simulink model "MotorController3"  (Simulink 10.1)
settings: Solver=ode5  StartTime=0.0  StopTime=100  FixedStep=5e-6  RelTol=1e-4  EnableMultiTasking=on
undefined symbols (not defined in the file): sigbuilder_block
libraries: simulink x5
settings Model: Creator=mf  LastModifiedBy=Lukas Bilal  SimulationMode=accelerator  ExtModeAutoUpdateStatusClock=off
settings Model: ModifiedHistory=|
  | Original Modell stammt von Martin Fränzle, Universität Oldenburg.
  | Erweiterung durch Stefan Disch, Universität Freiburg
settings DataIOCC: LimitDataPoints=on  SignalLoggingSaveFormat=ModelDataLogs  SaveOutput=off  SignalLogging=off  DSMLogging=off  SaveTime=off  SignalLoggingName=sigsOut
settings OptimizationCC: BooleanDataType=off  ExpressionDepthLimit=2147483647  InitFltsAndDblsToZero=on  SimCompilerOptimization=on
settings DebuggingCC: SaveWithParameterizedLinksMsg=none  SignalResolutionControl=TryResolveAllWithWarning  MultiTaskDSMMsg=warning  MultiTaskCondExecSysMsg=none  FcnCallInpInsideContextMsg=warning  StateNameClashWarn=warning
settings HardwareCC: TargetUnknown=on
settings SFSimCC: SimParseCustomCode=off
settings GRTTargetCC: TargetFcnLib=ansi_tfl_tmw.mat  ModelReferenceCompliant=off  MatFileLogging=off

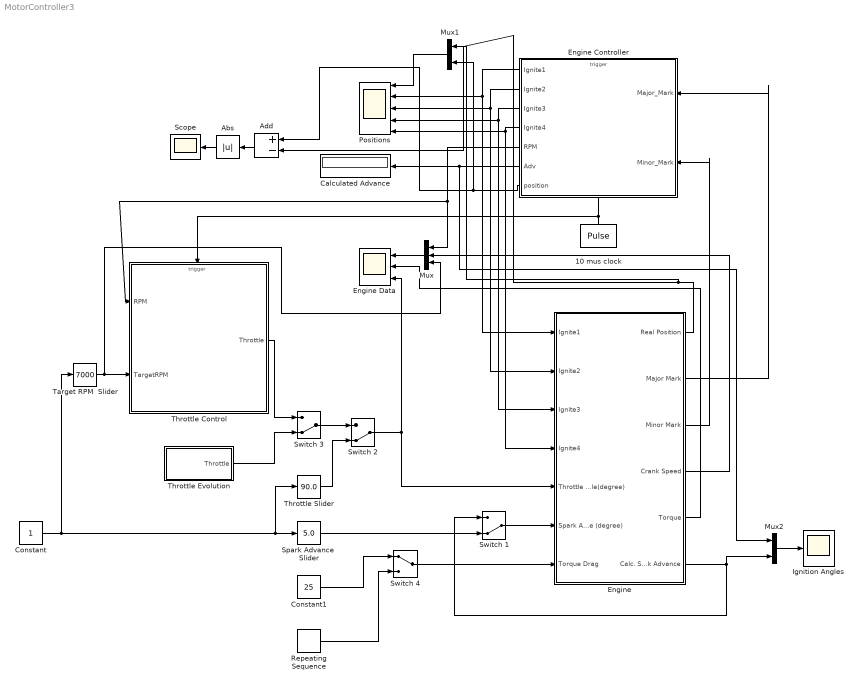
== system MotorController3 ==
  10 mus clock : DiscretePulseGenerator  PulseType=Time based  Period=1e-5  PulseWidth=50
  Abs : Abs
  Add : Sum  Inputs=+-
  Calculated Advance : Display
  Constant : Constant
  Constant1 : Constant  Value=25
  Engine : Subsystem
  Engine Controller : Stateflow chart  TreatAsAtomicUnit=on
  Engine Data : Scope  NumInputPorts=3
  Ignition Angles : Scope
  Mux : Mux  Inputs=3
  Mux1 : Mux  Inputs=2
  Mux2 : Mux  Inputs=2
  Positions : Scope  NumInputPorts=5
  Repeating Sequence : simulink/Sources/Repeating Sequence  rep_seq_t=[0 1 2 3 4 5 6]  rep_seq_y=[20 40 60 80 40 0 20]
  Scope : Scope
  Spark Advance  Slider : simulink/Math Operations/Slider Gain  gain=5.0  low=-15  high=60
  Switch 1 : ManualSwitch  CurrentSetting=0
  Switch 2 : ManualSwitch  CurrentSetting=0
  Switch 3 : ManualSwitch  CurrentSetting=0
  Switch 4 : ManualSwitch
  Target RPM  Slider : simulink/Math Operations/Slider Gain  gain=7000  low=800  high=7000
  Throttle Control : Stateflow chart  TreatAsAtomicUnit=on
  Throttle Evolution : Subsystem  Tag=STV Subsys  LoadFcn=sigbuilder_block('load');  StartFcn=sigbuilder_block('start');  StopFcn=sigbuilder_block('stop');  ClipboardFcn=sigbuilder_block('clipboard');  mask(Sigbuilder block){tuvar=[0:10]}
      mask help: Simulink:masks:SigbuilderBlock_MD
      mask init:
      | if ~strcmp(get_param(bdroot(gcbh),'SimulationStatus'),'stopped') tuvar = sigbuilder_block('maskInit'); end
      settings: CopyFcn=sigbuilder_block('copy');  DeleteFcn=sigbuilder_block('delete');  ModelCloseFcn=sigbuilder_block('modelClose');  PreSaveFcn=sigbuilder_block('preSave');  PauseFcn=sigbuilder_block('pause')  ContinueFcn=sigbuilder_block('continue')  NameChangeFcn=sigbuilder_block('namechange');  OpenFcn=sigbuilder_block('open',[54.75 146.25 550.5 390.75 ]);  CloseFcn=sigbuilder_block('close');
      mask Display: plot(0, 0, 100, 100,[2, 2, 32, 32, 2], [68, 8, 8, 68, 68],[32, 2], [38, 38], [32, 19, 2],[53, 60, 44], [32, 17, 17, 2],[16, 16, 31, 31]);txt = getActiveGroup(gcbh);text(2, 100, txt,'verticalAlignment', 'top');
  Throttle Slider : simulink/Math Operations/Slider Gain  gain=90.0  low=0  high=90
  wires:
  Engine Controller/3(Ignite3) -> Engine/3(Ignite3), Positions/4
  Engine Controller/2(Ignite2) -> Engine/2(Ignite2), Positions/3
  Engine Controller/1(Ignite1) -> Engine/1(Ignite1), Positions/2
  Engine Controller/4(Ignite4) -> Engine/4(Ignite4), Positions/5
  10 mus clock/1 -> Engine Controller/Trigger, Throttle Control/Trigger
  Engine Controller/5(RPM) -> Throttle Control/1(RPM), Mux/1
  Engine Controller/7(position) -> Mux1/2, Add/1
  Mux1/1 -> Positions/1
  Engine Controller/6(Adv) -> Calculated Advance/1, Mux2/1
  Switch 2/1 -> Engine Data/3, Engine/5(Throttle Angle(degree))
  Constant/1 -> Spark Advance  Slider/1, Throttle Slider/1, Target RPM  Slider/1
  Throttle Slider/1 -> Switch 2/2
  Spark Advance  Slider/1 -> Switch 1/2
  Mux2/1 -> Ignition Angles/1
  Mux/1 -> Engine Data/1
  Switch 3/1 -> Switch 2/1
  Throttle Evolution/1(Throttle) -> Switch 3/2
  Throttle Control/1(Throttle) -> Switch 3/1
  Target RPM  Slider/1 -> Throttle Control/2(TargetRPM), Mux/3
  Constant1/1 -> Switch 4/1
  Repeating Sequence/1 -> Switch 4/2
  Engine/6(" Calc. Spark Advance") -> Switch 1/1, Mux2/2
  Switch 1/1 -> Engine/6(Spark Advance (degree))
  Switch 4/1 -> Engine/7(Torque Drag)
  Engine/1(Real Position) -> Mux1/1, Add/2
  Engine/2(Major Mark) -> Engine Controller/1(Major_Mark)
  Engine/3(Minor Mark) -> Engine Controller/2(Minor_Mark)
  Engine/4(Crank Speed) -> Mux/2
  Engine/5(Torque) -> Engine Data/2
  Abs/1 -> Scope/1
  Add/1 -> Abs/1

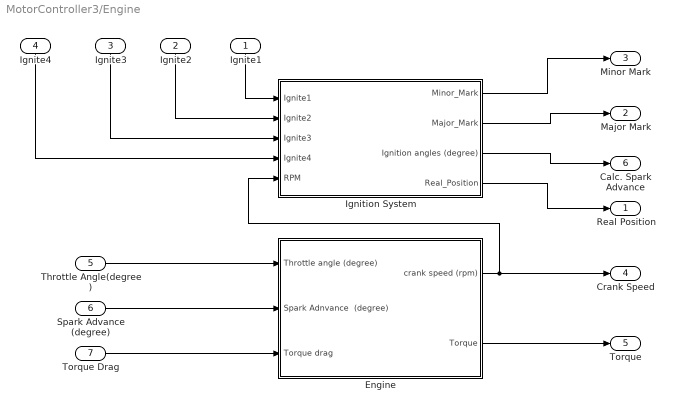
== system MotorController3/Engine ==
  Ignite1 : Inport
  Ignite2 : Inport  Port=2
  Ignite3 : Inport  Port=3
  Ignite4 : Inport  Port=4
  Throttle Angle(degree) : Inport  Port=5
  Spark Advance (degree) : Inport  Port=6
  Torque Drag : Inport  Port=7
  Engine : Subsystem
  Ignition System : Subsystem
  Real Position : Outport
  Major Mark : Outport  Port=2
  Minor Mark : Outport  Port=3
  Crank Speed : Outport  Port=4
  Torque : Outport  Port=5
  " Calc. Spark Advance" : Outport  Port=6
  wires:
  Ignite3/1 -> Ignition System/3(Ignite3)
  Ignite4/1 -> Ignition System/4(Ignite4)
  Ignite1/1 -> Ignition System/1(Ignite1)
  Ignite2/1 -> Ignition System/2(Ignite2)
  Throttle Angle(degree)/1 -> Engine/1(Throttle angle (degree))
  Engine/1(crank speed (rpm)) -> Ignition System/5(RPM), Crank Speed/1
  Ignition System/1(Minor_Mark) -> Minor Mark/1
  Ignition System/2(Major_Mark) -> Major Mark/1
  Ignition System/3(Ignition angles (degree)) -> " Calc. Spark Advance"/1
  Ignition System/4(Real_Position) -> Real Position/1
  Spark Advance (degree)/1 -> Engine/2(Spark Adnvance  (degree))
  Engine/2(Torque) -> Torque/1
  Torque Drag/1 -> Engine/3(Torque drag)

== system MotorController3/Throttle Evolution ==
  Demux : Demux  Tag=STV Demux  Outputs=1
      settings: DisplayOption=none
  FromWs : FromWorkspace  Tag=STV FromWs  VariableName=tuvar  SigBuilderData=DataTag0  VnvData=DataTag1
      SigBuilderData=|
      | common.afterFinalStr = 'Extrapolate'
      | common.sampleTime = 0
      | dataSet.timeRange = [0 14]
      | dataSet.name = 'Group 1'
      | sbobj.Groups.Name = 'Group 1'
      | sbobj.Groups.Signals.Name = 'Throttle'
      | sbobj.Groups.Signals.XData = [0 0.4 1.4 2.4 2.8 3.4 3.8 4.4 5.8 7 8 9.8 12 13.2 14]
      | sbobj.Groups.Signals.YData = [0.2 10 90.2 90 0.2 0.2 90.2 11.8 11.4 26.4 39.8 40.2 40.8 0 0]
      | sbobj.Groups.TimeRange = [0 14]
  Throttle : Outport  Tag=STV Outport
  wires:
  Demux/1 -> Throttle/1
  FromWs/1 -> Demux/1

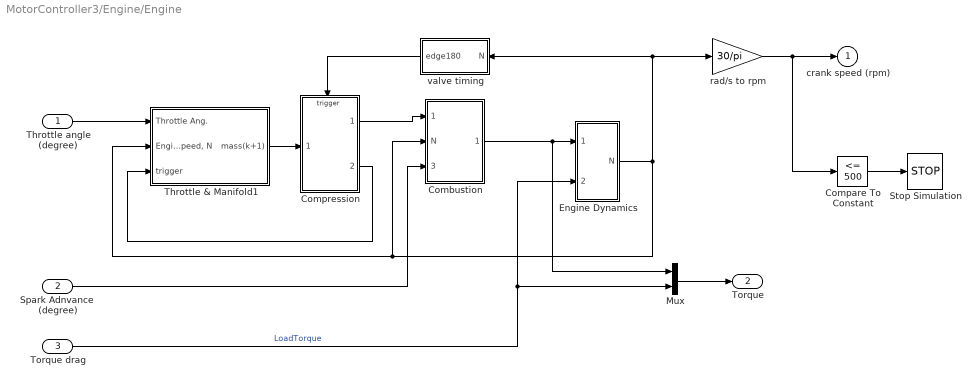
== system MotorController3/Engine/Engine ==
  Throttle angle (degree) : Inport  OutMin=0  OutMax=90  OutDataTypeStr=double
  Spark Adnvance  (degree) : Inport  Port=2
  Torque drag : Inport  Port=3  OutDataTypeStr=double
  Combustion : Subsystem
  Compare To Constant : simulink/Logic and Bit Operations/Compare To Constant  relop=<=  const=500  OutDataTypeStr=boolean
  Compression : Subsystem  TreatAsAtomicUnit=on
  Engine Dynamics : Subsystem
  Mux : Mux  Inputs=2
  Stop Simulation : Stop
  Throttle & Manifold1 : Subsystem
  rad/s to rpm : Gain  Gain=30/pi  SaturateOnIntegerOverflow=on  OutDataTypeStr=Inherit: Same as input  ParamDataTypeStr=Inherit: Same as input
  valve timing : Subsystem
  crank speed (rpm) : Outport  InitialOutput=0
  Torque : Outport  Port=2
  wires:
  valve timing/1(edge180) -> Compression/Trigger
  Compression/2(trigger) -> Throttle & Manifold1/3(trigger)
  Engine Dynamics/1(N) -> valve timing/1(N), rad/s to rpm/1, Throttle & Manifold1/2("Engine Speed, N"), Combustion/2(N)
  Compression/1(mass(k)) -> Combustion/1(Air Charge)
  Combustion/1(Torque) -> Engine Dynamics/1(Teng), Mux/1
  Mux/1 -> Torque/1
  Torque drag/1 -> Engine Dynamics/2(Tload), Mux/2  "LoadTorque"
  Throttle & Manifold1/1(mass(k+1)) -> Compression/1(mass(k+1))
  Throttle angle (degree)/1 -> Throttle & Manifold1/1(Throttle Ang.)
  rad/s to rpm/1 -> crank speed (rpm)/1, Compare To Constant/1
  Spark Adnvance  (degree)/1 -> Combustion/3(Spark Advance)
  Compare To Constant/1 -> Stop Simulation/1

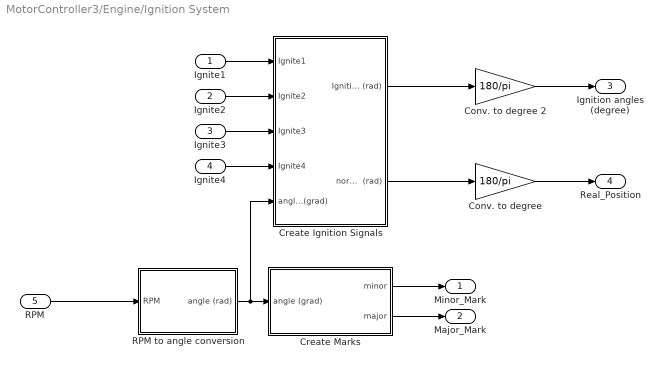
== system MotorController3/Engine/Ignition System ==
  Ignite1 : Inport  OutDataTypeStr=boolean
  Ignite2 : Inport  Port=2  OutDataTypeStr=boolean
  Ignite3 : Inport  Port=3  OutDataTypeStr=boolean
  Ignite4 : Inport  Port=4  OutDataTypeStr=boolean
  RPM : Inport  Port=5
  Conv. to degree : Gain  Gain=180/pi  SaturateOnIntegerOverflow=on  OutDataTypeStr=Inherit: Same as input  ParamDataTypeStr=Inherit: Same as input
  Conv. to degree 2 : Gain  Gain=180/pi  SaturateOnIntegerOverflow=on  OutDataTypeStr=Inherit: Same as input  ParamDataTypeStr=Inherit: Same as input
  Create Ignition Signals : Subsystem
  Create Marks : Subsystem
  RPM to angle conversion : Subsystem
  Minor_Mark : Outport
  Major_Mark : Outport  Port=2
  Ignition angles (degree) : Outport  Port=3
  Real_Position : Outport  Port=4
  wires:
  Create Marks/2(major) -> Major_Mark/1
  Create Marks/1(minor) -> Minor_Mark/1
  Ignite1/1 -> Create Ignition Signals/1(Ignite1)
  Ignite2/1 -> Create Ignition Signals/2(Ignite2)
  Ignite3/1 -> Create Ignition Signals/3(Ignite3)
  Ignite4/1 -> Create Ignition Signals/4(Ignite4)
  Create Ignition Signals/2(normalized angle  (rad)) -> Conv. to degree/1
  Create Ignition Signals/1(Ignition Advance  Angle (rad)) -> Conv. to degree 2/1
  RPM to angle conversion/1(angle (rad)) -> Create Marks/1(angle (grad)), Create Ignition Signals/5(angle (grad))
  Conv. to degree/1 -> Real_Position/1
  Conv. to degree 2/1 -> Ignition angles (degree)/1
  RPM/1 -> RPM to angle conversion/1(RPM)

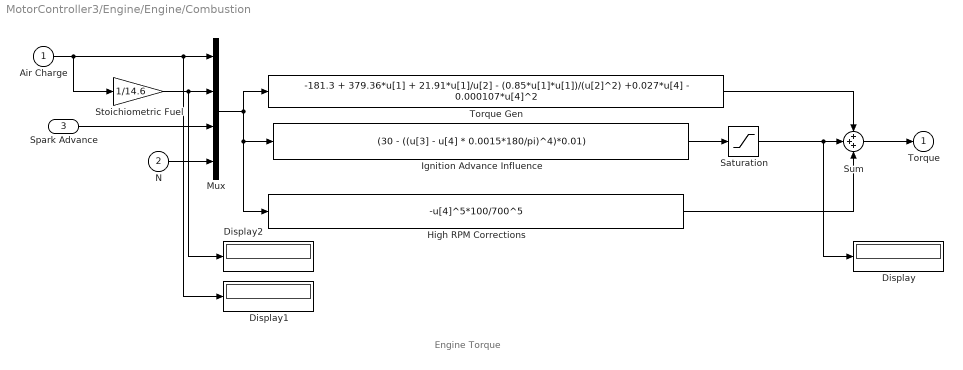
== system MotorController3/Engine/Engine/Combustion ==
  note: Engine Torque
  Air Charge : Inport
  N : Inport  Port=2
  Spark Advance : Inport  Port=3
  Display : Display
  Display1 : Display
  Display2 : Display
  High RPM Corrections : Fcn  Expr=-u[4]^5*100/700^5
  Ignition Advance Influence : Fcn  Expr=(30 - ((u[3] - u[4] * 0.0015*180/pi)^4)*0.01)
  Mux : Mux
  Saturation : Saturate  UpperLimit=150  LowerLimit=-150
  Stoichiometric Fuel : Gain  Gain=1/14.6  SaturateOnIntegerOverflow=on  OutDataTypeStr=Inherit: Same as input  ParamDataTypeStr=Inherit: Same as input
  Sum : Sum  Inputs=+++  InputSameDT=on  SaturateOnIntegerOverflow=on  OutDataTypeStr=Inherit: Same as first input
  Torque Gen : Fcn  Expr=-181.3 + 379.36*u[1] + 21.91*u[1]/u[2] - (0.85*u[1]*u[1])/(u[2]^2) +0.027*u[4] - 0.000107*u[4]^2
  Torque : Outport  InitialOutput=0
  wires:
  Sum/1 -> Torque/1
  Torque Gen/1 -> Sum/1
  Mux/1 -> Torque Gen/1, Ignition Advance Influence/1, High RPM Corrections/1
  Air Charge/1 -> Stoichiometric Fuel/1, Mux/1, Display1/1
  N/1 -> Mux/4
  Spark Advance/1 -> Mux/3
  Stoichiometric Fuel/1 -> Mux/2, Display2/1
  Ignition Advance Influence/1 -> Saturation/1
  High RPM Corrections/1 -> Sum/3
  Saturation/1 -> Sum/2, Display/1

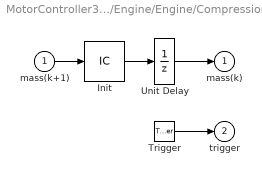
== system MotorController3/Engine/Engine/Compression ==
  mass(k+1) : Inport
  Trigger : TriggerPort  TriggerType=either  VariantControl=(inherit)  ShowOutputPort=on
  Init : InitialCondition  Value=0.152
  Unit Delay : UnitDelay  InitialCondition=0.152  SampleTime=-1  HasFrameUpgradeWarning=on
  mass(k) : Outport  InitialOutput=0.152
  trigger : Outport  Port=2  InitialOutput=-1
  wires:
  Trigger/1 -> trigger/1
  Unit Delay/1 -> mass(k)/1
  mass(k+1)/1 -> Init/1
  Init/1 -> Unit Delay/1

== system MotorController3/Engine/Engine/Engine Dynamics ==
  Teng : Inport
  Tload : Inport  Port=2
  "Inverse Inertia, 1/J" : Gain  Gain=1/0.15  SaturateOnIntegerOverflow=on  OutDataTypeStr=Inherit: Same as input  ParamDataTypeStr=Inherit: Same as input
  Sum : Sum  Inputs=+-  InputSameDT=on  SaturateOnIntegerOverflow=on  OutDataTypeStr=Inherit: Same as first input
  w = T/J w0 = 83.78 rad/s = 800 RPM : Integrator  InitialCondition=83.78
  N : Outport  InitialOutput=0
  wires:
  Tload/1 -> Sum/2
  Teng/1 -> Sum/1
  Sum/1 -> "Inverse Inertia, 1/J"/1
  w = T/J w0 = 83.78 rad/s = 800 RPM/1 -> N/1
  "Inverse Inertia, 1/J"/1 -> w = T/J w0 = 83.78 rad/s = 800 RPM/1

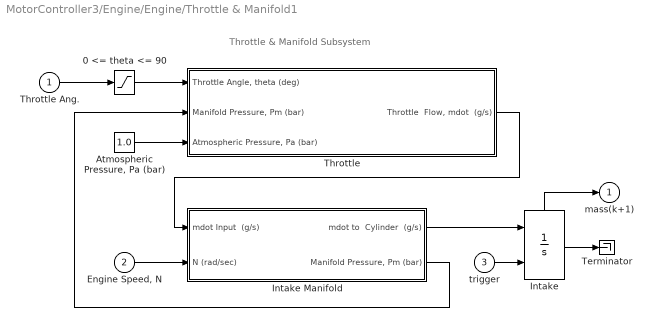
== system MotorController3/Engine/Engine/Throttle & Manifold1 ==
  note: Throttle & Manifold Subsystem
  Throttle Ang. : Inport
  "Engine Speed, N" : Inport  Port=2
  trigger : Inport  Port=3
  0 <= theta <= 90 : Saturate  UpperLimit=90  LowerLimit=0
  "Atmospheric Pressure, Pa (bar)" : Constant  Value=1.0
  Intake : Integrator  ExternalReset=either  ShowStatePort=on
  Intake Manifold : Subsystem
  Terminator : Terminator
  Throttle : Subsystem
  mass(k+1) : Outport  InitialOutput=0
  wires:
  0 <= theta <= 90/1 -> Throttle/1("Throttle Angle, theta (deg)")
  Throttle Ang./1 -> 0 <= theta <= 90/1
  Throttle/1("Throttle  Flow, mdot  (g/s)") -> Intake Manifold/1(mdot Input  (g/s))
  "Engine Speed, N"/1 -> Intake Manifold/2(N (rad/sec))
  Intake Manifold/2("Manifold Pressure, Pm (bar)") -> Throttle/2("Manifold Pressure, Pm (bar)")
  Intake Manifold/1(mdot to  Cylinder  (g/s)) -> Intake/1
  "Atmospheric Pressure, Pa (bar)"/1 -> Throttle/3("Atmospheric Pressure, Pa (bar) ")
  Intake/State -> mass(k+1)/1
  trigger/1 -> Intake/2
  Intake/1 -> Terminator/1

== system MotorController3/Engine/Engine/valve timing ==
  note: Rotational Velocity to Synchronized
      | Discrete Event Conversion
  N : Inport
  TDC and BDC detection : Subsystem
  positive edge to dual edge conversion : Subsystem  TreatAsAtomicUnit=on
  edge180 : Outport  InitialOutput=-1
  wires:
  N/1 -> TDC and BDC detection/1(N)  "rad/sec"
  positive edge to dual edge conversion/1(trigger) -> edge180/1
  TDC and BDC detection/1(trigger) -> positive edge to dual edge conversion/Trigger

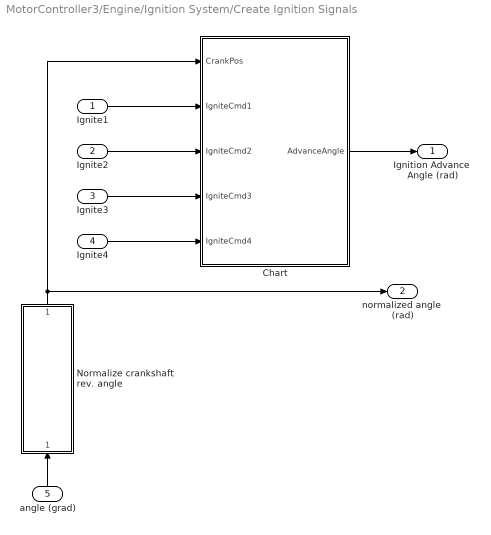
== system MotorController3/Engine/Ignition System/Create Ignition Signals ==
  Ignite1 : Inport
  Ignite2 : Inport  Port=2
  Ignite3 : Inport  Port=3
  Ignite4 : Inport  Port=4
  angle (grad) : Inport  Port=5
  Chart : Stateflow chart  TreatAsAtomicUnit=on
  Normalize crankshaft rev. angle : Subsystem
  Ignition Advance  Angle (rad) : Outport
  normalized angle  (rad) : Outport  Port=2
  wires:
  Normalize crankshaft rev. angle/1(Normalized to [0,4 pi)) -> Chart/1(CrankPos), normalized angle  (rad)/1
  angle (grad)/1 -> Normalize crankshaft rev. angle/1(Total  angle)
  Ignite1/1 -> Chart/2(IgniteCmd1)
  Chart/1(AdvanceAngle) -> Ignition Advance  Angle (rad)/1
  Ignite2/1 -> Chart/3(IgniteCmd2)
  Ignite3/1 -> Chart/4(IgniteCmd3)
  Ignite4/1 -> Chart/5(IgniteCmd4)

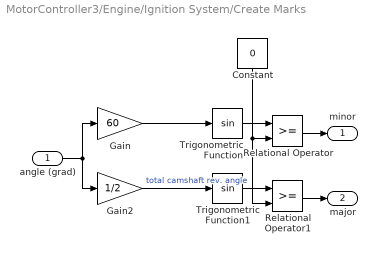
== system MotorController3/Engine/Ignition System/Create Marks ==
  angle (grad) : Inport
  Constant : Constant  Value=0
  Gain : Gain  Gain=60  SaturateOnIntegerOverflow=on  OutDataTypeStr=Inherit: Same as input  ParamDataTypeStr=Inherit: Same as input
  Gain2 : Gain  Gain=1/2  SaturateOnIntegerOverflow=on  OutDataTypeStr=Inherit: Same as input  ParamDataTypeStr=Inherit: Same as input
  Relational Operator : RelationalOperator  OutDataTypeStr=boolean  RndMeth=Nearest
  Relational Operator1 : RelationalOperator  OutDataTypeStr=boolean  RndMeth=Nearest
  Trigonometric Function : Trigonometry
  Trigonometric Function1 : Trigonometry
  minor : Outport
  major : Outport  Port=2
  wires:
  Constant/1 -> Relational Operator1/2, Relational Operator/2
  Gain/1 -> Trigonometric Function/1
  Gain2/1 -> Trigonometric Function1/1  "total camshaft rev. angle"
  angle (grad)/1 -> Gain2/1, Gain/1
  Relational Operator/1 -> minor/1
  Relational Operator1/1 -> major/1
  Trigonometric Function/1 -> Relational Operator/1
  Trigonometric Function1/1 -> Relational Operator1/1

== system MotorController3/Engine/Ignition System/RPM to angle conversion ==
  RPM : Inport
  Gain1 : Gain  Gain=2*pi  SaturateOnIntegerOverflow=on  OutDataTypeStr=Inherit: Same as input  ParamDataTypeStr=Inherit: Same as input
  Gain3 : Gain  Gain=1/60  SaturateOnIntegerOverflow=on  OutDataTypeStr=Inherit: Same as input  ParamDataTypeStr=Inherit: Same as input
  Total rev.s : Integrator
  angle (rad) : Outport
  wires:
  Gain3/1 -> Total rev.s/1
  Total rev.s/1 -> Gain1/1
  Gain1/1 -> angle (rad)/1  "total crankshaft rev. angle"
  RPM/1 -> Gain3/1

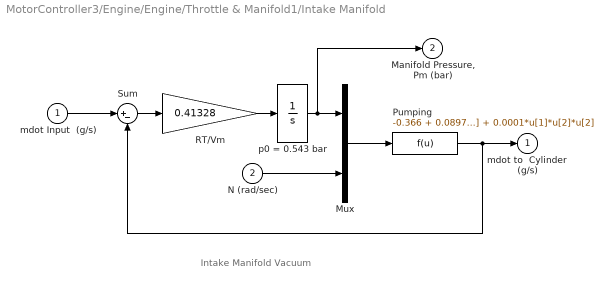
== system MotorController3/Engine/Engine/Throttle & Manifold1/Intake Manifold ==
  note: Intake Manifold Vacuum
  mdot Input  (g/s) : Inport
  N (rad/sec) : Inport  Port=2
  Mux : Mux  Inputs=2
  Pumping : Fcn  Expr=-0.366 + 0.08979*u[1]*u[2] - 0.0337*u[2]*u[1]*u[1] + 0.0001*u[1]*u[2]*u[2]
  RT/Vm : Gain  Gain=0.41328  SaturateOnIntegerOverflow=on  OutDataTypeStr=Inherit: Same as input  ParamDataTypeStr=Inherit: Same as input
  Sum : Sum  Inputs=|+-  InputSameDT=on  SaturateOnIntegerOverflow=on  OutDataTypeStr=Inherit: Same as first input
  p0 = 0.543 bar : Integrator  InitialCondition=.543
  mdot to  Cylinder  (g/s) : Outport  InitialOutput=0
  "Manifold Pressure, Pm (bar)" : Outport  Port=2  InitialOutput=0
  wires:
  mdot Input  (g/s)/1 -> Sum/1
  RT/Vm/1 -> p0 = 0.543 bar/1
  N (rad/sec)/1 -> Mux/2
  Mux/1 -> Pumping/1
  p0 = 0.543 bar/1 -> Mux/1, "Manifold Pressure, Pm (bar)"/1
  Sum/1 -> RT/Vm/1
  Pumping/1 -> Sum/2, mdot to  Cylinder  (g/s)/1

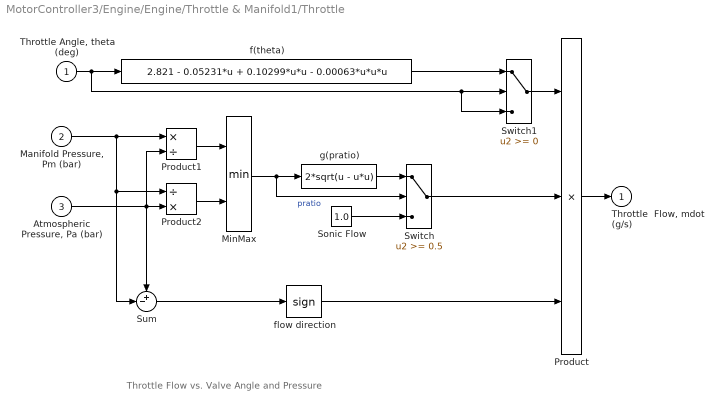
== system MotorController3/Engine/Engine/Throttle & Manifold1/Throttle ==
  note: Throttle Flow vs. Valve Angle and Pressure
  "Throttle Angle, theta (deg)" : Inport
  "Manifold Pressure, Pm (bar)" : Inport  Port=2
  "Atmospheric Pressure, Pa (bar) " : Inport  Port=3
  MinMax : MinMax  Inputs=2  InputSameDT=on  SaturateOnIntegerOverflow=on
  Product : Product  Inputs=3  InputSameDT=on  RndMeth=Zero  SaturateOnIntegerOverflow=on  OutDataTypeStr=Inherit: Same as first input
  Product1 : Product  Inputs=*/  InputSameDT=on  RndMeth=Zero  SaturateOnIntegerOverflow=on  OutDataTypeStr=Inherit: Same as first input
  Product2 : Product  Inputs=/*  InputSameDT=on  RndMeth=Zero  SaturateOnIntegerOverflow=on  OutDataTypeStr=Inherit: Same as first input
  "Sonic Flow " : Constant  Value=1.0
  Sum : Sum  Inputs=+-|  InputSameDT=on  SaturateOnIntegerOverflow=on  OutDataTypeStr=Inherit: Same as first input
  Switch : Switch  Threshold=0.5  SaturateOnIntegerOverflow=on  InputSameDT=on
  Switch1 : Switch  SaturateOnIntegerOverflow=on  InputSameDT=on
  f(theta) : Fcn  Expr=2.821 - 0.05231*u + 0.10299*u*u - 0.00063*u*u*u
  flow direction : Signum
  g(pratio) : Fcn  Expr=2*sqrt(u - u*u)
  "Throttle  Flow, mdot  (g/s)" : Outport  InitialOutput=0
  wires:
  "Manifold Pressure, Pm (bar)"/1 -> Sum/2, Product2/1, Product1/1
  Product2/1 -> MinMax/2
  Product1/1 -> MinMax/1
  "Atmospheric Pressure, Pa (bar) "/1 -> Sum/1, Product2/2, Product1/2
  g(pratio)/1 -> Switch/1
  "Sonic Flow "/1 -> Switch/3
  Switch/1 -> Product/2
  flow direction/1 -> Product/3
  Sum/1 -> flow direction/1
  MinMax/1 -> Switch/2, g(pratio)/1  "pratio"
  "Throttle Angle, theta (deg)"/1 -> f(theta)/1, Switch1/2, Switch1/3
  Product/1 -> "Throttle  Flow, mdot  (g/s)"/1
  Switch1/1 -> Product/1
  f(theta)/1 -> Switch1/1

== system MotorController3/Engine/Engine/valve timing/TDC and BDC detection ==
  note: Look for next top dead center.and
      | bottom dead center.
      | Produce two pulses per revolution.
  N : Inport
  Constant : Constant  Value=pi
  Get Crank Angle IC 0 : Integrator  ExternalReset=rising  ShowStatePort=on
  Relational Operator : RelationalOperator  RndMeth=Nearest  InputSameDT=on
  Terminator : Terminator
  trigger : Outport  InitialOutput=0
  wires:
  N/1 -> Get Crank Angle IC 0/1
  Relational Operator/1 -> trigger/1, Get Crank Angle IC 0/2
  Constant/1 -> Relational Operator/2
  Get Crank Angle IC 0/State -> Relational Operator/1
  Get Crank Angle IC 0/1 -> Terminator/1

== system MotorController3/Engine/Engine/valve timing/positive edge to dual edge conversion ==
  Trigger : TriggerPort  VariantControl=(inherit)
  Gain : Gain  Gain=-1  SaturateOnIntegerOverflow=on  OutDataTypeStr=Inherit: Same as input  ParamDataTypeStr=Inherit: Same as input
  Unit Delay : UnitDelay  InitialCondition=1  SampleTime=-1  HasFrameUpgradeWarning=on
  trigger : Outport  InitialOutput=-1
  wires:
  Unit Delay/1 -> Gain/1, trigger/1
  Gain/1 -> Unit Delay/1

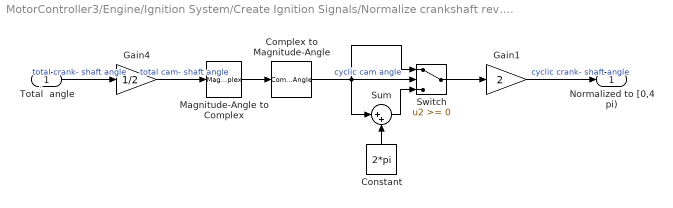
== system MotorController3/Engine/Ignition System/Create Ignition Signals/Normalize crankshaft rev. angle ==
  note: .
  Total  angle : Inport
  Complex to Magnitude-Angle : ComplexToMagnitudeAngle  Output=Angle
  Constant : Constant  Value=2*pi
  Gain1 : Gain  Gain=2  SaturateOnIntegerOverflow=on  OutDataTypeStr=Inherit: Same as input  ParamDataTypeStr=Inherit: Same as input
  Gain4 : Gain  Gain=1/2  SaturateOnIntegerOverflow=on  OutDataTypeStr=Inherit: Same as input  ParamDataTypeStr=Inherit: Same as input
  Magnitude-Angle to Complex : MagnitudeAngleToComplex  Input=Angle  ConstantPart=1
  Sum : Sum  Inputs=|++  SaturateOnIntegerOverflow=on
  Switch : Switch  SaturateOnIntegerOverflow=on
  Normalized to [0,4 pi) : Outport
  wires:
  Gain4/1 -> Magnitude-Angle to Complex/1  "total cam- shaft angle"
  Total  angle/1 -> Gain4/1  "total crank- shaft angle"
  Magnitude-Angle to Complex/1 -> Complex to Magnitude-Angle/1
  Complex to Magnitude-Angle/1 -> Sum/1, Switch/1, Switch/2  "cyclic cam angle"
  Sum/1 -> Switch/3
  Constant/1 -> Sum/2
  Switch/1 -> Gain1/1
  Gain1/1 -> Normalized to [0,4 pi)/1  "cyclic crank- shaft angle"

== stateflow chart Engine Controller ==
  settings: executeAtInitialization=1
  state Position [parallel]
    settings: executionOrder=1
    state FrequencyCounterMethode [parallel]
      settings: executionOrder=4
      state Clock [parallel]
        settings: executionOrder=1
        state Clock
        Position.FrequencyCounterMethode.Clock.Clock -> Position.FrequencyCounterMethode.Clock.Clock : clk [timeClock <  3e4]
            | {
            |   timeClock = timeClock + 1;
            | }  // Implementiert einfach
            |    // einen Timer.
      state Counter [parallel]
        settings: executionOrder=2
        state Counter
        Position.FrequencyCounterMethode.Counter.Counter -> Position.FrequencyCounterMethode.Counter.Counter [order 1] : [timeClock == 3e4]
            | {
            |   frequency_count =  1e5* frequency_counter/timeClock;
            |   timeClock = 0;
            |   frequency_counter = 0;
            | }
        Position.FrequencyCounterMethode.Counter.Counter -> Position.FrequencyCounterMethode.Counter.Counter [order 2] : [timeClock < 3e4 && hasChangedTo(Minor_Mark, 1)]
            | {
            |   frequency_counter  = frequency_counter + 1;  // Zählt die Zyklen
            | }
    state PositionCalculater [parallel]
      settings: executionOrder=3
      state ResetWithMajorMark [parallel]
        settings: executionOrder=1
        state MajoMarks
        MajoMarks -> MajoMarks : [hasChangedTo(Major_Mark, 1)] {
            |                                 position = 0;
            |                                 minormarks = 0;
            |                        }
      state PositionCalculater [parallel]
        settings: executionOrder=2
        state PositionCalculater/
          during: position = position +  60 * RPM *1e-6;
        Position.PositionCalculater.PositionCalculater.PositionCalculater -> Position.PositionCalculater.PositionCalculater.PositionCalculater : [hasChangedTo(Minor_Mark, 1)] {
            |  position = 6 * minormarks;
            | minormarks = minormarks + 1;
            |  }
    state FrequencyTimerMethode [parallel]
      settings: executionOrder=1
      state ClockStarter
      state FirstHigh
      state FirstLow
      (default) -> ClockStarter
      FirstHigh -> FirstLow [order 1] : [~Minor_Mark] / {cycles = cycles + 1;}
      FirstLow -> FirstLow [order 1] : [~Minor_Mark] / {cycles = cycles + 1;}
      ClockStarter -> FirstHigh : [Minor_Mark] /{cycles = 1;}
      FirstLow -> FirstHigh [order 2] : [Minor_Mark] {
          |   frequency_cycles = 1e5  * cycles;  // 1000, weil die Periodendauer 1/10^-3 s = 1000 s
          |   cycles = 0;
          |  }
      FirstHigh -> FirstHigh [order 2] : [Minor_Mark] /{cycles = cycles + 1;}  // Solange kein low kam, vergehen Zyklen
    state SparkAngles [parallel]
      settings: executionOrder=5
      state Engine1/
        during: Adv = RPM * 60 * 1e-6 * 1500;
      state Engine47
        during: Adv = RPM * 60 * 1e-6 * 1500;
      state HoldIgnite4
      state HoldIgnite3
      state HoldIgnite1
      state HoldIgnite2
      state Engine3/
        during: Adv = RPM * 60 * 1e-6 * 1500;
      state Engine2/
        during: Adv = RPM * 60 * 1e-6 * 1500;
      (default) -> Engine1
      HoldIgnite4 -> Engine1 : after(5, clk) {
          |   Ignite4 = 0;
          | }
      Engine47 -> HoldIgnite4 : [position >= 180 - Adv] {
          |   Ignite4 = 1;
          | }
      Engine1 -> HoldIgnite1 : [position >= 720 - Adv] {
          |   Ignite1 = 1;
          | }
      HoldIgnite3 -> Engine47 : after(5, clk) {
          |   Ignite3 = 0;
          | }
      Engine3 -> HoldIgnite3 : [position  >= 360 - Adv] {
          |   Ignite3 = 1;
          | }
      HoldIgnite1 -> Engine2 : after(50, clk) / {
          |   Ignite1 = 0;
          | }
      Engine2 -> HoldIgnite2 : [position >= 540 - Adv] {
          |   Ignite2 = 1;
          | }
      HoldIgnite2 -> Engine3 : after(5, clk) {
          |   Ignite2 = 0;
          | }
    state Evaluation [parallel]
      settings: executionOrder=2
      state EnableFrequency_cycles/
        RPM = frequency_count;
      state EnableFrequency_count/
        RPM = frequency_count;
      EnableFrequency_count -> EnableFrequency_cycles : [frequency_count < 2000]
      (default) -> EnableFrequency_cycles
      EnableFrequency_cycles -> EnableFrequency_count : [frequency_count > 2000]
  data: Major_Mark input boolean; Minor_Mark input boolean; Ignite1 output boolean; Ignite2 output boolean; Ignite3 output boolean; Ignite4 output boolean; RPM output double [0..] =1000; Adv output double [0..] =0; position output double [0..720]; frequency_count local double =0; frequency_cycles local boolean =0; cycles local double =0; minormarks local double =0; timeClock local double =0; frequency_counter local double
  events: clk input RISING_EDGE_EVENT

== stateflow chart Engine/Ignition System/Create Ignition Signals/Chart ==
  state Cylinder1 [parallel]
    settings: executionOrder=1
    note: Note: CrankPos is normalized to 0 ... 4*pi
    state WaitForIgnition /
      entry: adiabatic1 = 0+pi*15/180*ml('rand');
    state Pre_Ignite
    note: Ignition before 0
    note: Ignition after 0
    state Post_Ignite
    (default) -> Cylinder1.Pre_Ignite
    Cylinder1.Pre_Ignite -> Cylinder1.WaitForIgnition  : [(CrankPos>= 3*pi)]
    Cylinder1.Post_Ignite -> Cylinder1.Pre_Ignite : [(CrankPos>= pi) && (CrankPos <= pi+1)]
    Cylinder1.WaitForIgnition  -> (junction 95) : [(CrankPos >= adiabatic1 && CrankPos <= 0 + pi*15/180) || IgniteCmd1] /
    (junction 95) -> Cylinder1.Post_Ignite [order 1] : [CrankPos < pi]/
        | AdvanceAngle = -CrankPos;
    (junction 95) -> Cylinder1.Post_Ignite [order 2] : [CrankPos >= pi]/
        | AdvanceAngle = 4*pi-CrankPos;
  state Cylinder2 [parallel]
    settings: executionOrder=2
    note: Note: CrankPos is normalized to 0 ... 4*pi
    state WaitForIgnition /
      entry: adiabatic2 = pi+pi*15/180*ml('rand');
    state Pre_Ignite
    state Post_Ignite
    (default) -> Cylinder2.Pre_Ignite
    Cylinder2.Pre_Ignite -> Cylinder2.WaitForIgnition  : [(CrankPos>= 0) && (CrankPos <= pi)]
    Cylinder2.Post_Ignite -> Cylinder2.Pre_Ignite : [(CrankPos>= 2*pi) && CrankPos <= 2*pi+1]
    Cylinder2.WaitForIgnition  -> Cylinder2.Post_Ignite : [((CrankPos >= adiabatic2) && (CrankPos <= pi + pi*15/180)) || IgniteCmd2] /
        | AdvanceAngle = pi - CrankPos;
  state Cylinder4 [parallel]
    settings: executionOrder=4
    note: Note: CrankPos is normalized to 0 ... 4*pi
    state WaitForIgnition /
      entry: adiabatic4 = normalize(pi*3+pi*15/180*ml('rand'));
    state Pre_Ignite
    state Post_Ignite
    (default) -> Cylinder4.Pre_Ignite
    Cylinder4.Pre_Ignite -> Cylinder4.WaitForIgnition  : [(CrankPos>= 2*pi) && (CrankPos <= 3*pi)]
    Cylinder4.Post_Ignite -> Cylinder4.Pre_Ignite : [(CrankPos>= 0) && (CrankPos <= 1)]
    Cylinder4.WaitForIgnition  -> Cylinder4.Post_Ignite : [((CrankPos >= adiabatic4) && (CrankPos <= 3*pi + pi*15/180)) || IgniteCmd4] /
        | AdvanceAngle = pi*3 - CrankPos;
  state Cylinder3 [parallel]
    settings: executionOrder=3
    note: Note: CrankPos is normalized to 0 ... 4*pi
    state WaitForIgnition /
      entry: adiabatic3 = normalize(pi*2+pi*15/180*ml('rand'));
    state Pre_Ignite
    state Post_Ignite
    (default) -> Cylinder3.Pre_Ignite
    Cylinder3.Pre_Ignite -> Cylinder3.WaitForIgnition  : [(CrankPos>= pi) && (CrankPos<=2*pi)]
    Cylinder3.Post_Ignite -> Cylinder3.Pre_Ignite : [(CrankPos>= 3*pi) && CrankPos <= 3*pi+1]
    Cylinder3.WaitForIgnition  -> Cylinder3.Post_Ignite : [((CrankPos >= adiabatic3) && (CrankPos <= pi*2 + pi*15/180)) || IgniteCmd3] /
        | AdvanceAngle = pi*2 - CrankPos;
  state normangle = normalize(angle) [function]
    (default) -> (junction 120) : /*normalize the angle to [0,4*pi)*/
    (junction 120) -> (junction 119) [order 2] : [angle  < 0]
    (junction 120) -> (junction 121) [order 1] : [angle >= 4*pi]
    (junction 119) -> (junction 122) : {normangle = angle+4*pi;}
    (junction 121) -> (junction 124) : {normangle = angle-4*pi;}
    (junction 120) -> (junction 123) [order 3] : {normangle=angle;}
    (junction 122) -> (junction 123)
    (junction 124) -> (junction 123)
    (junction 123) -> (junction 125)
  data: adiabatic1 local double; adiabatic2 local double; adiabatic4 local double; adiabatic3 local double; angle function_input double; normangle function_output double; AdvanceAngle output double =0; CrankPos input double; IgniteCmd1 input double; pi constant double =3.14159265; IgniteCmd2 input double; IgniteCmd3 input double; IgniteCmd4 input double

== stateflow chart Throttle Control ==
  data: RPM input double; TargetRPM input double; Throttle output double [0..90] =0
  events: clk input RISING_EDGE_EVENT
